simulink model "untitled"  (R2021b)
settings: Solver=VariableStepAuto  StartTime=0.0  StopTime=2  RelTol=1e-3
libraries: dspstat3 x2, simulink x1
settings Model: Creator=riku3  LastModifiedBy=riku3
settings SolverCC: ZeroCrossAlgorithm=Adaptive
settings DebuggingCC: IgnoredZcDiagnostic=none

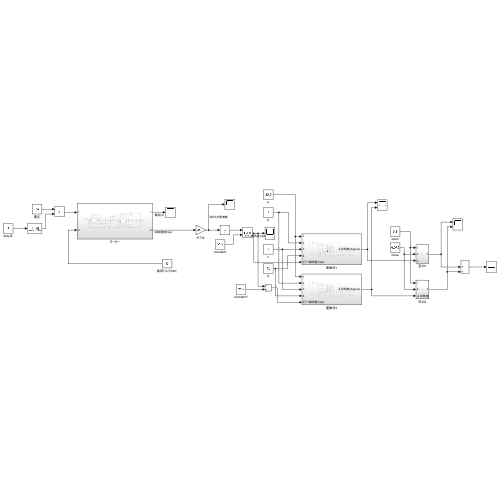
[thumbnail: Simulink's stored preview of the top-level diagram]
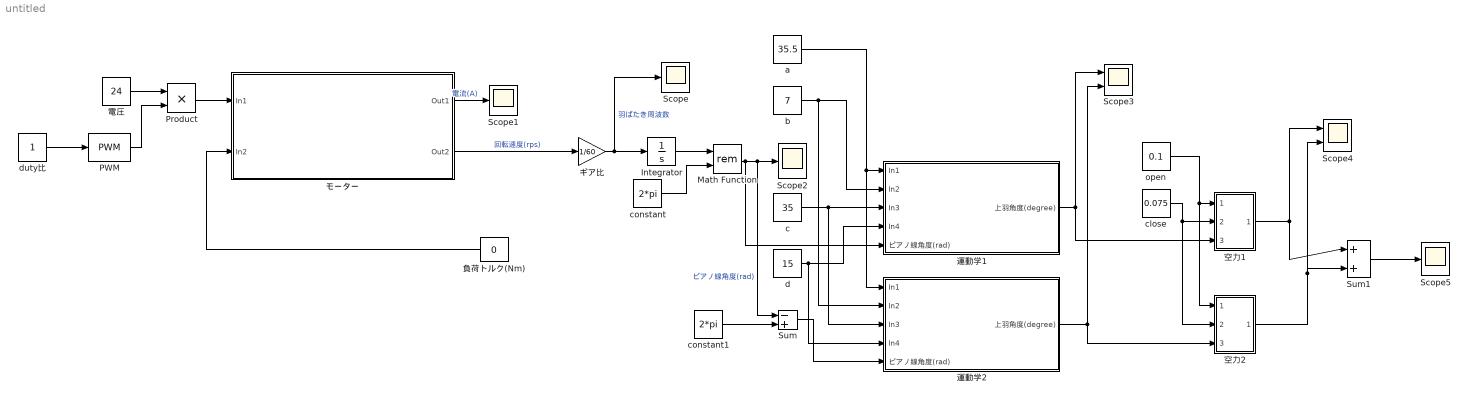
== system untitled ==
  Integrator : Integrator
  Math Function : Math  Operator=rem  SaturateOnIntegerOverflow=on
  PWM : simulink/Discontinuities/PWM  DisableCoverage=on  Period=1/20e3  DisallowZeroDutyCycle=off  RunAtFixedTimeIntervals=off  SampleTime=0.1
  Product : Product  Inputs=**
  Scope{,1..2,5} (4 alike) : Scope
  Scope3 : Scope  NumInputPorts=2
  Scope4 : Scope  NumInputPorts=2
  Sum : Sum  Inputs=-+
  Sum1 : Sum  Inputs=|++
  a : Constant  Value=35.5
  b : Constant  Value=7
  c : Constant  Value=35
  close : Constant  Value=0.075
  constant : Constant  Value=2*pi
  constant1 : Constant  Value=2*pi
  d : Constant  Value=15
  duty比 : Constant
  open : Constant  Value=0.1
  ギア比 : Gain  Gain=1/60
  モーター : Subsystem
  空力1 : Subsystem
  空力2 : Subsystem
  負荷トルク(Nm) : Constant  Value=0
  運動学1 : Subsystem
  運動学2 : Subsystem
  電圧 : Constant  Value=24
  wires:
  運動学2/1(上羽角度(degree)) -> 空力2/3(上羽角度(degree)), Scope3/2
  Sum/1 -> 運動学2/5(ピアノ線角度(rad))
  運動学1/1(上羽角度(degree)) -> 空力1/3(In3), Scope3/1
  電圧/1 -> Product/1
  ギア比/1 -> Scope/1, Integrator/1  "羽ばたき周波数"
  c/1 -> 運動学2/3(In3), 運動学1/3(In3)
  Integrator/1 -> Math Function/1
  constant/1 -> Math Function/2
  constant1/1 -> Sum/2
  モーター/1(Out1) -> Scope1/1  "電流(A)"
  負荷トルク(Nm)/1 -> モーター/2(In2)
  Product/1 -> モーター/1(In1)
  PWM/1 -> Product/2
  duty比/1 -> PWM/1
  d/1 -> 運動学1/4(In4), 運動学2/4(In4)
  b/1 -> 運動学2/2(In2), 運動学1/2(In2)
  a/1 -> 運動学2/1(In1), 運動学1/1(In1)
  Math Function/1 -> Sum/1, Scope2/1, 運動学1/5(ピアノ線角度(rad))  "ピアノ線角度(rad)"
  モーター/2(Out2) -> ギア比/1  "回転速度(rps)"
  open/1 -> 空力2/1(In1), 空力1/1(In1)
  close/1 -> 空力2/2(In2), 空力1/2(In2)
  空力1/1(Out1) -> Sum1/1, Scope4/1
  空力2/1(Out1) -> Sum1/2, Scope4/2
  Sum1/1 -> Scope5/1

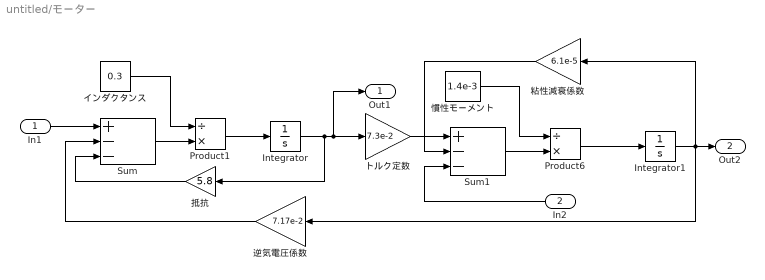
== system untitled/モーター ==
  In1 : Inport
  In2 : Inport  Port=2
  Integrator : Integrator
  Integrator1 : Integrator  InitialCondition=600
  Product1 : Product  Inputs=/*
  Product6 : Product  Inputs=/*
  Sum : Sum  Inputs=+--
  Sum1 : Sum  Inputs=+--
  インダクタンス : Constant  Value=0.3
  トルク定数 : Gain  Gain=7.3e-2
  慣性モーメント : Constant  Value=1.4e-3
  抵抗 : Gain  Gain=5.8
  粘性減衰係数 : Gain  Gain=6.1e-5
  逆気電圧係数 : Gain  Gain=7.17e-2
  Out1 : Outport
  Out2 : Outport  Port=2
  wires:
  慣性モーメント/1 -> Product6/1
  トルク定数/1 -> Sum1/1
  粘性減衰係数/1 -> Sum1/2
  In2/1 -> Sum1/3
  抵抗/1 -> Sum/3
  逆気電圧係数/1 -> Sum/2
  In1/1 -> Sum/1
  Sum1/1 -> Product6/2
  Product1/1 -> Integrator/1
  インダクタンス/1 -> Product1/1
  Sum/1 -> Product1/2
  Product6/1 -> Integrator1/1
  Integrator1/1 -> 逆気電圧係数/1, 粘性減衰係数/1, Out2/1
  Integrator/1 -> Out1/1, トルク定数/1, 抵抗/1

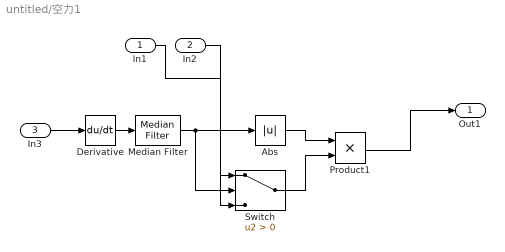
== system untitled/空力1 ==
  In1 : Inport
  In2 : Inport  Port=2
  In3 : Inport  Port=3
  Abs : Abs
  Derivative : Derivative
  Median Filter : dspstat3/Median Filter  WindowLength=50  SimulateUsing=Interpreted execution
      settings: SourceProductBaseCode=DS
  Product1 : Product
  Switch : Switch  Criteria=u2 > Threshold
  Out1 : Outport
  wires:
  Abs/1 -> Product1/1
  Switch/1 -> Product1/2
  In3/1 -> Derivative/1
  Product1/1 -> Out1/1
  In1/1 -> Switch/1
  Median Filter/1 -> Switch/2, Abs/1
  In2/1 -> Switch/3
  Derivative/1 -> Median Filter/1

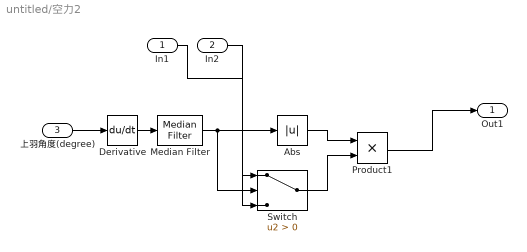
== system untitled/空力2 ==
  In1 : Inport
  In2 : Inport  Port=2
  上羽角度(degree) : Inport  Port=3
  Abs : Abs
  Derivative : Derivative
  Median Filter : dspstat3/Median Filter  WindowLength=50  SimulateUsing=Interpreted execution
      settings: SourceProductBaseCode=DS
  Product1 : Product
  Switch : Switch  Criteria=u2 > Threshold
  Out1 : Outport
  wires:
  Abs/1 -> Product1/1
  Switch/1 -> Product1/2
  上羽角度(degree)/1 -> Derivative/1
  Product1/1 -> Out1/1
  In1/1 -> Switch/1
  Median Filter/1 -> Switch/2, Abs/1
  In2/1 -> Switch/3
  Derivative/1 -> Median Filter/1

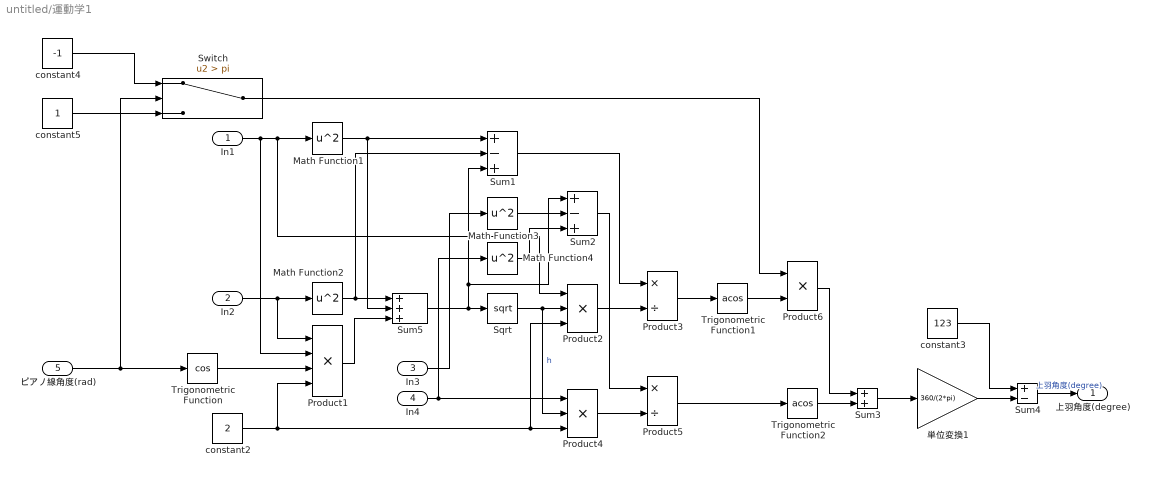
== system untitled/運動学1 ==
  In1 : Inport
  In2 : Inport  Port=2
  In3 : Inport  Port=3
  In4 : Inport  Port=4
  ピアノ線角度(rad) : Inport  Port=5
  Math Function{1..4} (4 alike) : Math  Operator=square  SaturateOnIntegerOverflow=on
  Product1 : Product  Inputs=****
  Product2 : Product  Inputs=***
  Product3 : Product  Inputs=*/
  Product4 : Product  Inputs=***
  Product5 : Product  Inputs=*/
  Product6 : Product  Inputs=**
  Sqrt : Sqrt  SaturateOnIntegerOverflow=on
  Sum1 : Sum  Inputs=+-+
  Sum2 : Sum  Inputs=+-+
  Sum3 : Sum
  Sum4 : Sum  Inputs=+-
  Sum5 : Sum  Inputs=+++
  Switch : Switch  Criteria=u2 > Threshold  Threshold=pi
  Trigonometric Function : Trigonometry  Operator=cos
  Trigonometric Function1 : Trigonometry  Operator=acos
  Trigonometric Function2 : Trigonometry  Operator=acos
  constant2 : Constant  Value=2
  constant3 : Constant  Value=123
  constant4 : Constant  Value=-1
  constant5 : Constant
  単位変換1 : Gain  Gain=360/(2*pi)
  上羽角度(degree) : Outport
  wires:
  ピアノ線角度(rad)/1 -> Switch/2, Trigonometric Function/1
  constant5/1 -> Switch/3
  constant3/1 -> Sum4/1
  単位変換1/1 -> Sum4/2
  Product1/1 -> Sum5/3
  Sum5/1 -> Sum2/1, Sum1/3, Sqrt/1
  Sum2/1 -> Product5/1
  Product4/1 -> Product5/2
  Product2/1 -> Product3/2
  Sum1/1 -> Product3/1
  Sum3/1 -> 単位変換1/1
  Trigonometric Function2/1 -> Sum3/2
  Trigonometric Function1/1 -> Product6/2
  Sum4/1 -> 上羽角度(degree)/1  "上羽角度(degree)"
  Math Function4/1 -> Sum2/3
  Switch/1 -> Product6/1
  Trigonometric Function/1 -> Product1/3
  Product5/1 -> Trigonometric Function2/1
  In3/1 -> Math Function3/1
  constant4/1 -> Switch/1
  Math Function3/1 -> Sum2/2
  Product3/1 -> Trigonometric Function1/1
  Product6/1 -> Sum3/1
  Math Function2/1 -> Sum1/2, Sum5/1
  In4/1 -> Product4/1, Math Function4/1
  constant2/1 -> Product2/3, Product4/3, Product1/4
  Math Function1/1 -> Sum1/1, Sum5/2
  In2/1 -> Math Function2/1, Product1/1
  In1/1 -> Product2/1, Math Function1/1, Product1/2
  Sqrt/1 -> Product2/2, Product4/2  "h"

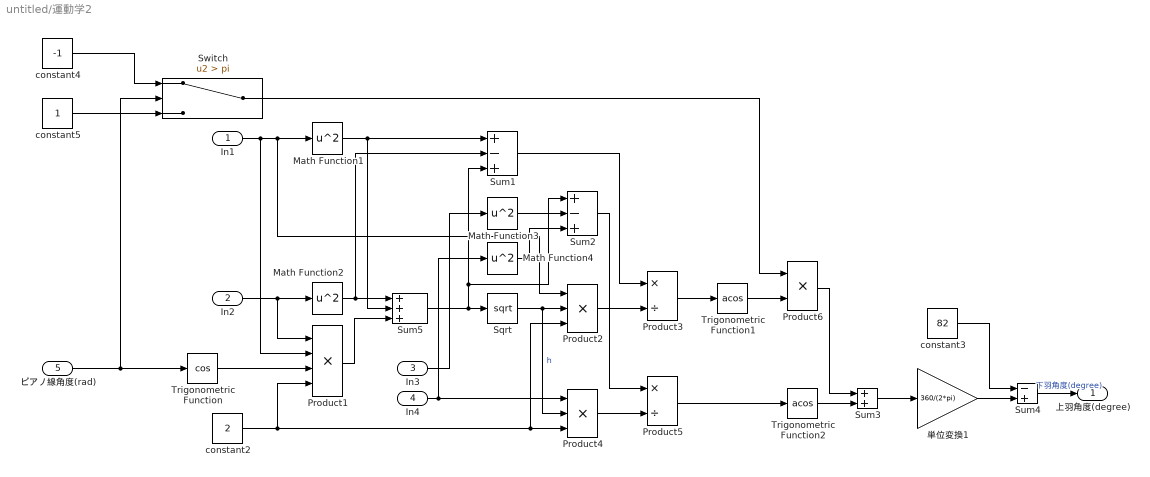
== system untitled/運動学2 ==
  In1 : Inport
  In2 : Inport  Port=2
  In3 : Inport  Port=3
  In4 : Inport  Port=4
  ピアノ線角度(rad) : Inport  Port=5
  Math Function{1..4} (4 alike) : Math  Operator=square  SaturateOnIntegerOverflow=on
  Product1 : Product  Inputs=****
  Product2 : Product  Inputs=***
  Product3 : Product  Inputs=*/
  Product4 : Product  Inputs=***
  Product5 : Product  Inputs=*/
  Product6 : Product  Inputs=**
  Sqrt : Sqrt  SaturateOnIntegerOverflow=on
  Sum1 : Sum  Inputs=+-+
  Sum2 : Sum  Inputs=+-+
  Sum3 : Sum
  Sum4 : Sum  Inputs=-+
  Sum5 : Sum  Inputs=+++
  Switch : Switch  Criteria=u2 > Threshold  Threshold=pi
  Trigonometric Function : Trigonometry  Operator=cos
  Trigonometric Function1 : Trigonometry  Operator=acos
  Trigonometric Function2 : Trigonometry  Operator=acos
  constant2 : Constant  Value=2
  constant3 : Constant  Value=82
  constant4 : Constant  Value=-1
  constant5 : Constant
  単位変換1 : Gain  Gain=360/(2*pi)
  上羽角度(degree) : Outport
  wires:
  Product4/1 -> Product5/2
  constant3/1 -> Sum4/1
  単位変換1/1 -> Sum4/2
  Math Function2/1 -> Sum5/1, Sum1/2
  constant5/1 -> Switch/3
  Sum2/1 -> Product5/1
  Product1/1 -> Sum5/3
  Trigonometric Function2/1 -> Sum3/2
  Sum3/1 -> 単位変換1/1
  Sum1/1 -> Product3/1
  Product2/1 -> Product3/2
  Sum4/1 -> 上羽角度(degree)/1  "下羽角度(degree)"
  Math Function4/1 -> Sum2/3
  Trigonometric Function1/1 -> Product6/2
  In1/1 -> Product2/1, Math Function1/1, Product1/2
  Switch/1 -> Product6/1
  Trigonometric Function/1 -> Product1/3
  Product5/1 -> Trigonometric Function2/1
  Sum5/1 -> Sum2/1, Sum1/3, Sqrt/1
  constant4/1 -> Switch/1
  Math Function3/1 -> Sum2/2
  In3/1 -> Math Function3/1
  Product3/1 -> Trigonometric Function1/1
  In4/1 -> Math Function4/1, Product4/1
  Product6/1 -> Sum3/1
  constant2/1 -> Product2/3, Product4/3, Product1/4
  ピアノ線角度(rad)/1 -> Trigonometric Function/1, Switch/2
  In2/1 -> Product1/1, Math Function2/1
  Math Function1/1 -> Sum5/2, Sum1/1
  Sqrt/1 -> Product4/2, Product2/2  "h"
